simulink model "PV_wind_bat_DC_Microgrid"  (R2013a)
settings: Solver=ode23tb  StartTime=0  StopTime=3  RelTol=1e-3
undefined symbols (not defined in the file): c1, c2, c3, c4, c5, c6, DiscIntNeverNeededParam, fdesignblkfcn, gcbh, Hydride, Metal, Nickel
libraries: dspsigops x53, powerlib x33, powerlib_extras x6, electricdrivelib x1, dsparch4 x1, simulink x1
(part 1 of 2)
settings Model: Creator=cbhende  LastModifiedBy=user
settings SolverCC: ZeroCrossControl=DisableAll
settings DataIOCC: SaveFormat=StructureWithTime  SignalLoggingSaveFormat=ModelDataLogs  SaveOutput=off  SignalLogging=off  SaveTime=off
settings OptimizationCC: InlineParams=on  ExpressionDepthLimit=2147483647  InitFltsAndDblsToZero=on  EfficientFloat2IntCast=on
settings DebuggingCC: FcnCallInpInsideContextMsg=UseLocalSettings  StrictBusMsg=Warning
settings GRTTargetCC: CombineOutputUpdateFcns=off  GRTInterface=on

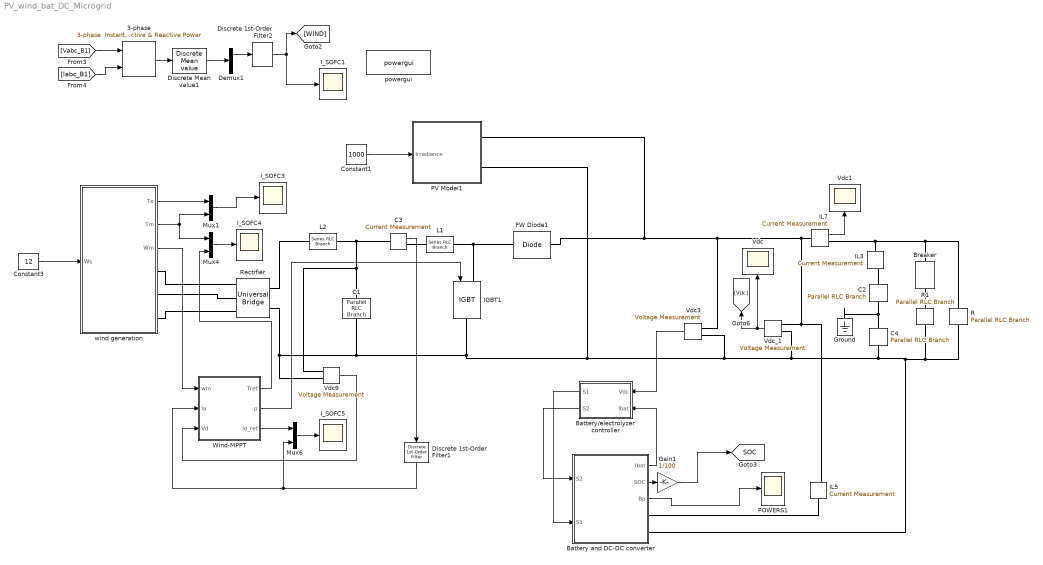
== system PV_wind_bat_DC_Microgrid ==
  "3-phase " : powerlib_extras/Measurements/3-phase  Instantaneous  Active & Reactive Power
  Battery and DC-DC converter : Subsystem
  Battery/electrolyzer controller : Subsystem
  Breaker : powerlib/Elements/Breaker  BreakerResistance=0.01  InitialState=0  SnubberResistance=1e6  SnubberCapacitance=inf  SwitchingTimes=[1 5]  External=off  Measurements=None  MoreParameters=off  NoBreakLoop=off
  C1 : powerlib/Elements/Parallel RLC Branch  LConnTagsString=a  RConnTagsString=__new0  BranchType=C  Resistance=1.0  Inductance=1.0  SetiL0=off  InitialCurrent=0  Capacitance=1000e-06  Setx0=off  InitialVoltage=0  Measurements=None
  C2 : powerlib/Elements/Parallel RLC Branch  LConnTagsString=a  RConnTagsString=__new0  BranchType=C  Resistance=1.0  Inductance=1.0  SetiL0=off  InitialCurrent=0  Capacitance=2200e-06*2  Setx0=off  InitialVoltage=0  Measurements=None
  C3 : powerlib/Measurements/Current Measurement  PhasorSimulation=off  OutputType=Complex  PSBequivalent=0
  C4 : powerlib/Elements/Parallel RLC Branch  LConnTagsString=a  RConnTagsString=__new0  BranchType=C  Resistance=1.0  Inductance=1.0  SetiL0=off  InitialCurrent=0  Capacitance=2200e-06*2  Setx0=off  InitialVoltage=0  Measurements=None
  Constant1 : Constant  Value=1000
  Constant3 : Constant  Value=12
  Demux1 : Demux  Outputs=2
  Discrete 1st-Order Filter1 : powerlib_extras/Discrete  Control Blocks/Discrete 1st-Order Filter  FilterType=Lowpass  Tc=100e-3  Ts=20e-6  Initialize=off  Vac_Init=[0.8 -25 60]  Vdc_Init=-0.4  PlotResponse=off  param1=[1 500 0.1]
  Discrete 1st-Order Filter2 : powerlib_extras/Discrete  Control Blocks/Discrete 1st-Order Filter  FilterType=Lowpass  Tc=100e-3  Ts=20e-6  Initialize=off  Vac_Init=[0.8 -25 60]  Vdc_Init=-0.4  PlotResponse=off  param1=[1 500 0.1]
  Discrete Mean value1 : powerlib_extras/Discrete Measurements/Discrete  Mean value  Freq=50  Vinit=0  Ts=20e-6
  FW Diode1 : powerlib/Power Electronics/Diode  Ron=0.01  Lon=0  Vf=0.8  IC=0  UseSnubber=off  Rs=100  Cs=0.1e-6  Measurements=off
  Gain1 : Gain  Gain=1/100
  Ground : powerlib/Elements/Ground  LConnTagsString=a
  IGBT1 : powerlib/Power Electronics/IGBT  Ron=0.001  Lon=0  Vf=1  Tf=1e-6  Tt=2e-6  IC=0  Rs=1e5  Cs=inf  Measurements=off
  IL3 : powerlib/Measurements/Current Measurement  PhasorSimulation=off  OutputType=Complex  PSBequivalent=0
  IL5 : powerlib/Measurements/Current Measurement  PhasorSimulation=off  OutputType=Complex  PSBequivalent=0
  IL7 : powerlib/Measurements/Current Measurement  PhasorSimulation=off  OutputType=Complex  PSBequivalent=0
  I_SOFC{1,3..5} (4 alike) : Scope
      I_SOFC1 settings: TimeRange=1.5  YMin=6213.5  YMax=6222  SaveName=w  SampleTime=100e-6
      I_SOFC3 settings: TimeRange=0.04  YMin=3400  YMax=3675  SaveName=Vdc  SampleInput=on  SampleTime=100e-6
      I_SOFC4 settings: TimeRange=0.04  YMin=3400  YMax=3675  SaveName=Vdc1  SampleInput=on  SampleTime=100e-6
      I_SOFC5 settings: TimeRange=0.04  YMin=3400  YMax=3675  SaveName=Vdc2  SampleInput=on  SampleTime=100e-6
  L1 : powerlib/Elements/Series RLC Branch  LConnTagsString=__new0  RConnTagsString=__new0  BranchType=L  Resistance=1.0  Inductance=2e-3  SetiL0=off  InitialCurrent=0  Capacitance=1.0  Setx0=off  InitialVoltage=0  Measurements=None
  L2 : powerlib/Elements/Series RLC Branch  LConnTagsString=__new0  RConnTagsString=__new0  BranchType=L  Resistance=1.0  Inductance=2e-3  SetiL0=off  InitialCurrent=0  Capacitance=1.0  Setx0=off  InitialVoltage=0  Measurements=None
  Mux1 : Mux  Inputs=2
  Mux4 : Mux  Inputs=2
  Mux6 : Mux  Inputs=2
  POWERS1 : Scope
      settings: TimeRange=1.5  YMin=-4410  YMax=-4260  SaveName=power1
  PV Model1 : Subsystem  mask{Isc=8.01, Voc=36.90, Im=7.10, Vm=30.3, ns=22}
      mask prompts: Isc "Short-Circuit Current"; Voc "Open-Circuit Voltage"; Im "Current at Pmax"; Vm "Voltage at Pmax"; ns "Number of Modules connected in series"
      mask init:
      | % calculation of PV module parameters
      | % limitation: constant temperature
      | Ns = round(Voc/0.61); % default number of cells in series
      | Vt = 26e-3; % thermal voltage
      | G = Isc/1000; % irradiation to short-circuit current gain
      | Vmpc = Vm/Ns; % cell voltage at rated Pmax
      | Vocc = Voc/Ns; % cell open-circuit voltage
      | Rmpp = Vmpc/Im; % cell load resistance at Pmax
      | %
      | Rp = 100*Vocc/Isc; % initial value for Rp
      | Vdm = Vocc; % initial value for Vdm
      | %
      | % iterative solution for model parameters: Io, Rs, Rp
      | for i=1:10
      | %
      |  Idm = Isc - Im - Vdm/Rp; % pn-junction (diode) current at MPP
      |  Io = (Isc-Vocc/Rp)/(exp(Vocc/Vt)-1); % pn-junction reverse saturation current
      |  Vdm = Vt*log(Idm/Io+1); % pn-junction (diode) voltage at MPP
      |  Rs = (Vdm-Vmpc)/Im; % cell series resistance
      |  Rd = (Rmpp - Rs)*Rp/(Rp-Rmpp+Rs); % diode incremental resistance at MPP
      |  Idm = Vt/Rd; % diode current at MPP based on incremental resistance
      |  Rp = Vdm/(Isc-Im-Idm); % cell parallel resistance
      | %
      | end
      | %
  R : powerlib/Elements/Parallel RLC Branch  LConnTagsString=a  RConnTagsString=__new0  BranchType=R  Resistance=400  Inductance=1.0  SetiL0=off  InitialCurrent=0  Capacitance=2200e-06*2  Setx0=off  InitialVoltage=0  Measurements=None
  R1 : powerlib/Elements/Parallel RLC Branch  LConnTagsString=a  RConnTagsString=__new0  BranchType=R  Resistance=200  Inductance=1.0  SetiL0=off  InitialCurrent=0  Capacitance=2200e-06*2  Setx0=off  InitialVoltage=0  Measurements=None
  Rectifier : powerlib/Power Electronics/Universal Bridge  Arms=3  SnubberResistance=100  SnubberCapacitance=0.1e-6  Device=Diodes  Ron=1e-3  Lon=0  ForwardVoltages="[  0.8  0.8  ]"  ForwardVoltage=.8  GTOparameters=[ 10e-6 , 20e-6 ]  IGBTparameters=[ 1e-6 , 2e-6 ]  Measurements=Device currents  Measurements_2=None  converterType=Rectifier
  Vdc : Scope
      settings: YMin=658  YMax=678  SaveName=V_dc  SampleInput=on  SampleTime=100e-6
  Vdc1 : Scope
      settings: YMin=658  YMax=677  SaveName=V_dc1  SampleInput=on  SampleTime=100e-6
  Vdc3 : powerlib/Measurements/Voltage Measurement  Tag=PoWeRsYsTeMmEaSuReMeNt  PhasorSimulation=off  OutputType=Magnitude  PSBequivalent=0
  Vdc9 : powerlib/Measurements/Voltage Measurement  Tag=PoWeRsYsTeMmEaSuReMeNt  PhasorSimulation=off  OutputType=Magnitude  PSBequivalent=0
  Vdc_1 : powerlib/Measurements/Voltage Measurement  Tag=PoWeRsYsTeMmEaSuReMeNt  PhasorSimulation=off  OutputType=Magnitude  PSBequivalent=0
  Wind-MPPT : Subsystem
  powergui : powerlib/powergui  SimulationMode=Discrete  SolverType=Tustin  SampleTime=20e-6  frequency=60  SPID=off  DisableSnubberDevices=off  DisableRonSwitches=off  DisableVfSwitches=off  SwTol=0  Interpol=off  DisplayEquations=off  frequencyindice=0  Pbase=100e6  ErrMax=1e-4  Iterations=50  UnitsV=kV  UnitsW=MW  FunctionMessages=off  echomessages=off  HookPort=off  EnableUseOfTLC=off  x0status=blocks  RestoreLinks=warning  ResistiveCurrentMeasurement=off  Frange=[0:2:500]  Ylog=off  Xlog=on  ShowGrid=off  save=off  variable=ZData  structure=psbbridges_str  ZoomFFT=on  StartTime=2.5  cycles=1  DisplayStyle=2  fundamental=50  FreqAxis=on  MaxFrequency=5000  frequencyindicesteady=1  RmsSteady=1  display=off  Ts=0  methode=off
  wind generation : Subsystem
  tag scope: SOC=global
  wires:
  Battery/electrolyzer controller/1(S1) -> Battery and DC-DC converter/2(S1)
  Battery/electrolyzer controller/2(S2) -> Battery and DC-DC converter/1(S2)
  Battery and DC-DC converter/1(Ibat) -> Battery/electrolyzer controller/2(Ibat)
  Battery and DC-DC converter/2(SOC) -> Gain1/1
  Vdc3/1 -> Battery/electrolyzer controller/1(Vdc)
  Vdc_1/1 -> Vdc/1, [Vdc]
  Battery and DC-DC converter/3(Bp) -> POWERS1/1
  Gain1/1 -> [SOC]
  Constant1/1 -> PV Model1/1(Irradiance)
  wind generation/2(Tm) -> Mux4/1, Mux1/2
  Wind-MPPT/1(Tref) -> Mux4/2
  wind generation/1(Te) -> Mux1/1
  wind generation/3(Wm) -> Wind-MPPT/1(wm)
  Constant3/1 -> wind generation/1(Ws)
  C3/1 -> Discrete 1st-Order Filter1/1
  Mux1/1 -> I_SOFC3/1
  Mux4/1 -> I_SOFC4/1
  Wind-MPPT/2(p) -> IGBT1/1
  Vdc9/1 -> Wind-MPPT/3(Vd)
  Discrete 1st-Order Filter1/1 -> Wind-MPPT/2(Ia), Mux6/2
  Mux6/1 -> I_SOFC5/1
  Wind-MPPT/3(Id_ref) -> Mux6/1
  [Vabc_B1] -> "3-phase "/1
  Discrete Mean value1/1 -> Demux1/1
  [Iabc_B1] -> "3-phase "/2
  "3-phase "/1 -> Discrete Mean value1/1
  Demux1/1 -> Discrete 1st-Order Filter2/1
  Discrete 1st-Order Filter2/1 -> [WIND], I_SOFC1/1
  IL7/1 -> Vdc1/1
  connections:
  IL3/RConn1 -- C2/LConn1
  IL5/RConn1 -- PV Model1/RConn1 -- FW Diode1/RConn1 -- Vdc3/LConn1 -- IL7/LConn1 -- Vdc_1/LConn1
  C1/RConn1 -- PV Model1/RConn2 -- R/RConn1 -- R1/RConn1 -- Battery and DC-DC converter/RConn2 -- C4/RConn1 -- Vdc_1/LConn2 -- Vdc3/LConn2 -- IGBT1/RConn1 -- Vdc9/LConn2 -- Rectifier/RConn2
  Battery and DC-DC converter/RConn1 -- IL5/LConn1
  IL7/RConn1 -- R/LConn1 -- Breaker/LConn1 -- IL3/LConn1
  C4/LConn1 -- Ground/LConn1 -- C2/RConn1
  C3/LConn1 -- L2/RConn1 -- Vdc9/LConn1 -- C1/LConn1
  L1/RConn1 -- FW Diode1/LConn1 -- IGBT1/LConn1
  wind generation/RConn2 -- Rectifier/LConn2
  wind generation/RConn1 -- Rectifier/LConn1
  wind generation/RConn3 -- Rectifier/LConn3
  Rectifier/RConn1 -- L2/LConn1
  C3/RConn1 -- L1/LConn1
  R1/LConn1 -- Breaker/RConn1

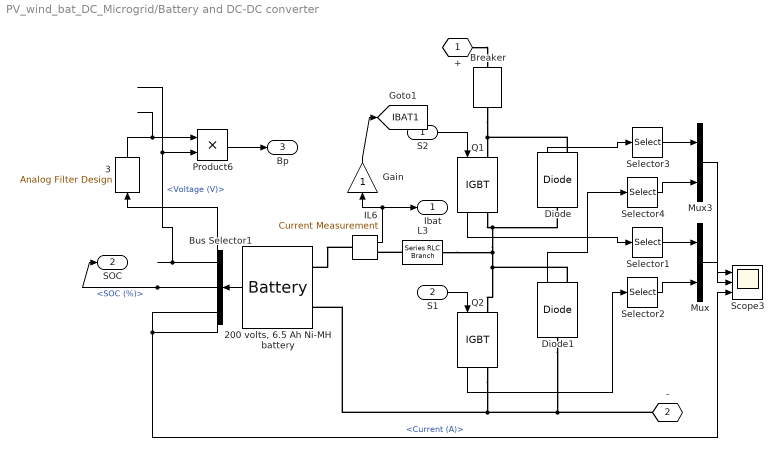
== system PV_wind_bat_DC_Microgrid/Battery and DC-DC converter ==
  S2 : Inport
  S1 : Inport  Port=2
  "200 volts, 6.5 Ah Ni-MH battery " : electricdrivelib/Extra Sources/Battery  BatType=Nickel-Metal-Hydride  ShowDetailedParameters=off  NomV=300  NomQ=50  SOC=60  PresetModel=on  MaxQ=53.8462  FullV=353.3898  Dis_rate=10  R=0.06  Normal_OP=48.0769  expZone="[325.4237            10]"  Dis_Char=off  current=[6.5 13 32.5]  Units=Time  Batt_Tr=30
  3 : dsparch4/Analog Filter Design  method=Butterworth  filttype=Lowpass  N=8  Wlo=pi*50  Whi=80  Rp=2  Rs=40
  Breaker : powerlib/Elements/Breaker  BreakerResistance=0.01  InitialState=1  SnubberResistance=1e6  SnubberCapacitance=inf  SwitchingTimes=[15 ]  External=off  Measurements=None  MoreParameters=off  NoBreakLoop=off
  Bus Selector1 : BusSelector  OutputSignals=Voltage (V),SOC (%),Current (A)
  Diode : powerlib/Power Electronics/Diode  Ron=0.001  Lon=0  Vf=0.8  IC=0  UseSnubber=off  Rs=500  Cs=250e-9  Measurements=on
  Diode1 : powerlib/Power Electronics/Diode  Ron=0.001  Lon=0  Vf=0.8  IC=0  UseSnubber=off  Rs=500  Cs=250e-9  Measurements=on
  Gain : Gain
  IL6 : powerlib/Measurements/Current Measurement  PhasorSimulation=off  OutputType=Complex  PSBequivalent=0
  L3 : powerlib/Elements/Series RLC Branch  LConnTagsString=__new0  RConnTagsString=__new0  BranchType=L  Resistance=1.0  Inductance=5e-3  SetiL0=off  InitialCurrent=0  Capacitance=1.0  Setx0=off  InitialVoltage=0  Measurements=None
  Mux : Mux  Inputs=2
  Mux3 : Mux  Inputs=2
  Product6 : Product  RndMeth=Zero
  Q1 : powerlib/Power Electronics/IGBT  Ron=0.001  Lon=0  Vf=1  Tf=1e-6  Tt=2e-6  IC=0  Rs=1e5  Cs=inf  Measurements=on
  Q2 : powerlib/Power Electronics/IGBT  Ron=0.001  Lon=0  Vf=1  Tf=1e-6  Tt=2e-6  IC=0  Rs=1e5  Cs=inf  Measurements=on
  Scope3 : Scope  NumInputPorts=3
      settings: TimeRange=0.1  YMin=0~0~-36  YMax=37.5~35~-23  SaveName=V2X  SampleInput=on  SampleTime=10e-6
  Selector{1..4} (4 alike) : Selector  InputPortWidth=2  IndexOptions=Index vector (dialog)  Indices=1  OutputSizes=1
  + : PMIOPort  Tag=PMCPort  Port=1  Side=Right
  - : PMIOPort  Tag=PMCPort  Port=2  Side=Right
  Ibat : Outport
  SOC : Outport  Port=2
  Bp : Outport  Port=3
  tag scope: IBAT1=global
  wires:
  "200 volts, 6.5 Ah Ni-MH battery "/1 -> Bus Selector1/1
  Bus Selector1/1 -> Product6/2  "<Voltage (V)>"
  Bus Selector1/2 -> SOC/1  "<SOC (%)>"
  Bus Selector1/3 -> Scope3/3, 3/1  "<Current (A)>"
  Product6/1 -> Bp/1
  Q1/1 -> Selector1/1
  Q2/1 -> Selector2/1
  Selector1/1 -> Mux/1
  Selector2/1 -> Mux/2
  Selector3/1 -> Mux3/1
  Selector4/1 -> Mux3/2
  Diode/1 -> Selector3/1
  Diode1/1 -> Selector4/1
  Mux/1 -> Scope3/1
  Mux3/1 -> Scope3/2
  S2/1 -> Q1/1
  S1/1 -> Q2/1
  IL6/1 -> Ibat/1, Gain/1
  3/1 -> Product6/1
  Gain/1 -> [IBAT1]
  connections:
  IL6/LConn1 -- "200 volts, 6.5 Ah Ni-MH battery "/LConn1
  "200 volts, 6.5 Ah Ni-MH battery "/LConn2 -- Q2/RConn1 -- -/RConn1 -- Diode1/LConn1
  +/RConn1 -- Breaker/LConn1
  Breaker/RConn1 -- Diode/RConn1 -- Q1/LConn1
  Q2/LConn1 -- Diode1/RConn1 -- L3/RConn1 -- Diode/LConn1 -- Q1/RConn1
  L3/LConn1 -- IL6/RConn1

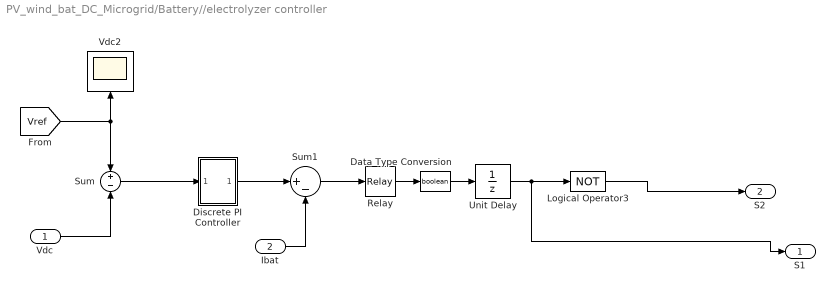
== system PV_wind_bat_DC_Microgrid/Battery//electrolyzer controller ==
  Vdc : Inport
  Ibat : Inport  Port=2
  Data Type Conversion : DataTypeConversion  OutDataTypeStr=boolean  RndMeth=Simplest  SaturateOnIntegerOverflow=on
  Discrete PI Controller : Subsystem  AncestorBlock=|  DialogController=POWERSYS.PowerSysDialog  mask(Discrete PI Controller){Kp=3, Ki=180, Par_Limits=[100  -100], Init=0, Ts=20e-6}
      | powerlib_extras/Discrete 
      | Control Blocks/Discrete
      | PI Controller
      mask prompts: Kp "Proportional gain (Kp):"; Ki "Integral gain (Ki):"; Par_Limits "Output limits: [ Upper   Lower ]"; Init "Output initial value:"; Ts "Sample time:"
      mask help: This block implements a discrete PI controller.
      mask init:
      | UpperLimit=Par_Limits(1);
      | LowerLimit=Par_Limits(2);
      | power_initmask();
      mask Help: This block is part of a subset of blocks in the Extras library that does not have documentation associated with it, other than the block mask description.
      mask Display: disp('PI');
  Logical Operator3 : Logic  Operator=NOT
  Relay : Relay  OnSwitchValue=1  OffSwitchValue=-1  OutDataTypeStr=Inherit: Inherit via back propagation
  Sum : Sum  Inputs=+-  SaturateOnIntegerOverflow=on  InputSameDT=on  OutDataTypeStr=Inherit: Same as first input
  Sum1 : Sum  Inputs=|+-  InputSameDT=on
  Unit Delay : UnitDelay  SampleTime=-1
  Vdc2 : Scope
      settings: YMin=654.997  YMax=655  SaveName=V_dc3  SampleInput=on  SampleTime=100e-6
  S1 : Outport
  S2 : Outport  Port=2
  wires:
  Vdc/1 -> Sum/2
  Logical Operator3/1 -> S2/1
  Discrete PI Controller/1(Out) -> Sum1/1
  Sum/1 -> Discrete PI Controller/1(Error)
  Relay/1 -> Data Type Conversion/1
  Ibat/1 -> Sum1/2
  Sum1/1 -> Relay/1
  Data Type Conversion/1 -> Unit Delay/1
  [Vref] -> Sum/1, Vdc2/1
  Unit Delay/1 -> S1/1, Logical Operator3/1

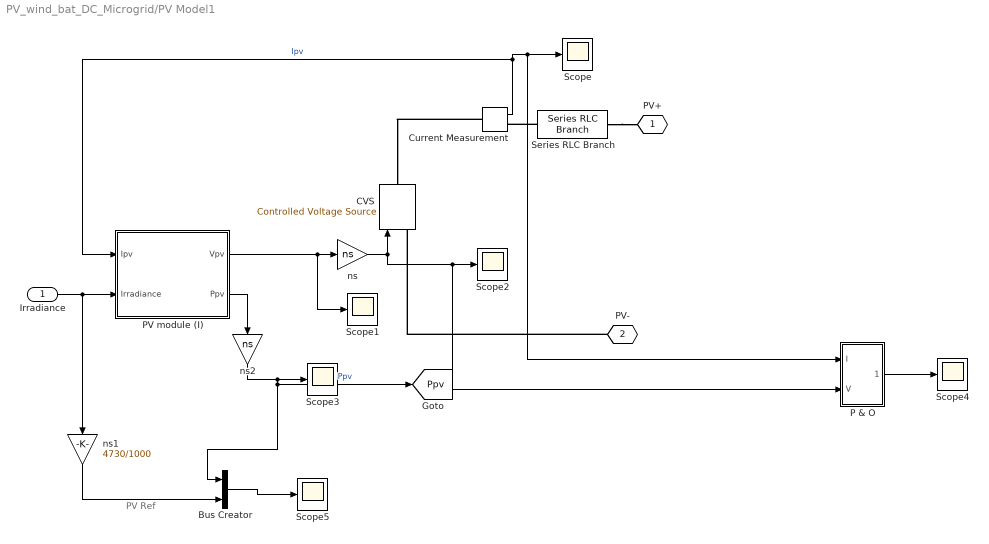
== system PV_wind_bat_DC_Microgrid/PV Model1 ==
  note: PV Ref
  Irradiance : Inport
  Bus Creator : BusCreator  Inputs=2
  CVS : powerlib/Electrical Sources/Controlled Voltage Source  Initialize=on  Source_Type=DC  Amplitude=0  Phase=0  Frequency=0  Measurements=None
  Current Measurement : powerlib/Measurements/Current Measurement  PhasorSimulation=off  OutputType=Complex  PSBequivalent=0
  P & O : Subsystem
  PV module (I) : Subsystem
  Scope{,1..5} (6 alike) : Scope
      Scope settings: YMin=3.3  YMax=3.355
      Scope1 settings: SaveName=ScopeData2
      Scope2 settings: YMin=653  YMax=668  SaveName=ScopeData3
      Scope3 settings: YMin=4645  YMax=4695  SaveName=ScopeData4
      Scope4 settings: YMin=609.9  YMax=674.1  SaveName=ScopeData28
      Scope5 settings: YMin=4710  YMax=4733  SaveName=ScopeData42
  Series RLC Branch : powerlib/Elements/Series RLC Branch  LConnTagsString=__new0  RConnTagsString=__new0  BranchType=R  Resistance=0.00001  Inductance=1e-3  SetiL0=off  InitialCurrent=0  Capacitance=1e-6  Setx0=off  InitialVoltage=0  Measurements=None
  ns : Gain  Gain=ns
  ns1 : Gain  Gain=4730/1000
  ns2 : Gain  Gain=ns
  PV+ : PMIOPort  Tag=PMCPort  Port=1  Side=Right
  PV- : PMIOPort  Tag=PMCPort  Port=2  Side=Right
  tag scope: Ppv=global
  wires:
  ns2/1 -> [Ppv], Bus Creator/1, Scope3/1  "Ppv"
  ns/1 -> CVS/1, Scope2/1, P & O/2(V)
  PV module (I)/2(Ppv) -> ns2/1
  Irradiance/1 -> PV module (I)/2(Irradiance), ns1/1
  Current Measurement/1 -> PV module (I)/1(Ipv), Scope/1, P & O/1(I)  "Ipv"
  PV module (I)/1(Vpv) -> Scope1/1, ns/1
  P & O/1(Vref) -> Scope4/1
  ns1/1 -> Bus Creator/2
  Bus Creator/1 -> Scope5/1
  connections:
  Series RLC Branch/LConn1 -- Current Measurement/RConn1
  Current Measurement/LConn1 -- CVS/RConn1
  PV-/RConn1 -- CVS/LConn1
  Series RLC Branch/RConn1 -- PV+/RConn1

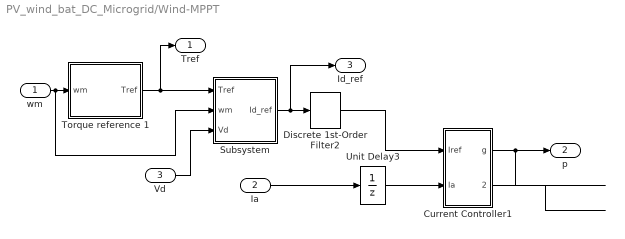
== system PV_wind_bat_DC_Microgrid/Wind-MPPT ==
  wm : Inport
  Ia : Inport  Port=2
  Vd : Inport  Port=3
  Current Controller1 : Subsystem  mask{h=0.1}
      mask prompts: h "Hysteresis band (A)"
      mask help: Hysteresis Current Controller
      mask Display: plot(0,0,100,100,[45,45],[35,65],[55,55],[35,65],[45,65],[65,65],[35,55],[35,35])
  Discrete 1st-Order Filter2 : powerlib_extras/Discrete  Control Blocks/Discrete 1st-Order Filter  FilterType=Lowpass  Tc=100e-3  Ts=20e-6  Initialize=off  Vac_Init=[0.8 -25 60]  Vdc_Init=-0.4  PlotResponse=off  param1=[1 500 0.1]
  Subsystem : Subsystem
  Torque reference 1 : Subsystem
  Unit Delay3 : UnitDelay  SampleTime=-1
  Tref : Outport
  p : Outport  Port=2
  Id_ref : Outport  Port=3
  wires:
  Unit Delay3/1 -> Current Controller1/2(Ia)
  Torque reference 1/1(Tref) -> Tref/1, Subsystem/1(Tref)
  Subsystem/1(Id_ref) -> Discrete 1st-Order Filter2/1, Id_ref/1
  Discrete 1st-Order Filter2/1 -> Current Controller1/1(Iref)
  Current Controller1/1(g) -> p/1
  wm/1 -> Torque reference 1/1(wm), Subsystem/2(wm)
  Vd/1 -> Subsystem/3(Vd)
  Ia/1 -> Unit Delay3/1
  Current Controller1/2(error1) -> ?

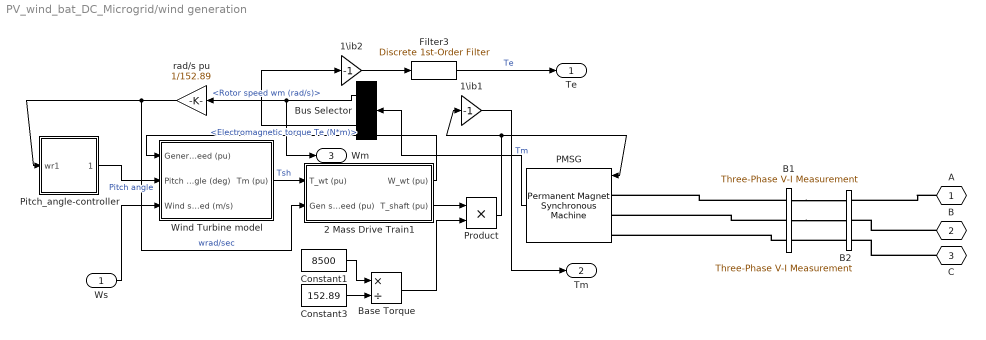
== system PV_wind_bat_DC_Microgrid/wind generation ==
  Ws : Inport
  1\ib1 : Gain  Gain=-1  SaturateOnIntegerOverflow=on  OutDataTypeStr=Inherit: Same as input  ParamDataTypeStr=Inherit: Same as input
  1\ib2 : Gain  Gain=-1  SaturateOnIntegerOverflow=on  OutDataTypeStr=Inherit: Same as input  ParamDataTypeStr=Inherit: Same as input
  2 Mass Drive Train1 : Subsystem
  B1 : powerlib/Measurements/Three-Phase V-I Measurement  VoltageMeasurement=phase-to-ground  SetLabelV=on  LabelV=Vabc_B1  Vpu=off  VpuLL=off  CurrentMeasurement=yes  SetLabelI=on  LabelI=Iabc_B1  Ipu=off  Pbase=100e6  Vbase=500e3  OutputType=Magnitude  PhasorSimulation=off  PSBequivalent=0
  "B2 " : powerlib/Measurements/Three-Phase V-I Measurement  VoltageMeasurement=no  SetLabelV=on  LabelV=Vabc_B2  Vpu=off  VpuLL=off  CurrentMeasurement=no  SetLabelI=on  LabelI=Iabc_B2  Ipu=off  Pbase=100e6  Vbase=500e3  OutputType=Magnitude  PhasorSimulation=off  PSBequivalent=0
  Base Torque : Product  Inputs=*/  RndMeth=Zero
  Bus Selector : BusSelector  OutputSignals=Rotor speed wm (rad/s),Electromagnetic torque Te (N*m)
  Constant1 : Constant  Value=8500
  Constant3 : Constant  Value=152.89
  Filter3 : powerlib_extras/Discrete  Control Blocks/Discrete 1st-Order Filter  FilterType=Lowpass  Tc=1e-3  Ts=20e-6  Initialize=off  Vac_Init=[0.8 -25 60]  Vdc_Init=-0.4  PlotResponse=off  param1=[1 500 0.1]
  PMSG : powerlib/Machines/Permanent Magnet Synchronous Machine  NbPhases=3  FluxDistribution=Sinusoidal  RotorType=Round  MechanicalLoad=Torque Tm  PresetModel=No  ShowDetailedParameters=on  Resistance=0.425  Inductance=8.5e-3  dqInductances=[0.0082 0.0082]  La=0.000835  MachineConstant=Flux linkage established by magnets (V.s)  Flux=0.433  VoltageCst=392.6876  TorqueCst=3.2475  Flat=120  Mechanical=[0.01197 0.001189 5]  PolePairs=5  InitialConditions=[0,0, 0,0]  InitialConditions5ph=[0 0 0 0 0 0]  TsPowergui=0  TsBlock=-1  RefAngle=90 degrees behind phase A axis (modified Park)
  Pitch_angle-controller : Subsystem
  Product : Product  RndMeth=Zero
  Wind Turbine model : Subsystem  AncestorBlock=DRlib/Wind Generation/Wind Turbine  DialogController=POWERSYS.PowerSysDialog  mask(Wind Turbine){Pnom=8.5e3, Pelec_base=8.5e3/0.9, wind_base=12, P_wind_base=0.8, speed_nom=1, pitch_angle=0, DisplayTurbChar=off, c1_c6=[0.51763          116          0.4            5           21     0.006795], cp_nom=0.48, lambda_nom=8.1}
      mask prompts: Pnom "Nominal mechanical output power (W):"; Pelec_base "Base power of the electrical generator (VA):"; wind_base "Base wind speed (m/s):"; P_wind_base "Maximum power at base wind speed (pu of nominal mechanical power):"; speed_nom "Base rotational speed (p.u. of base generator speed):"; pitch_angle "Pitch angle beta to display wind-turbine power characteristics (beta >=0)  (deg):"; DisplayTurbChar "Display wind turbine power characteristics"
      mask help:
      | This block implements a variable pitch wind turbine model. The performance coefficient Cp of the turbine is the mechanical output power of the turbine divided by wind power and a function of wind speed, rotational speed, and pitch angle (beta). Cp reaches its maximum value at zero beta. Select the wind-turbine power characteristics display to plot the turbine characteristics at the specified pitch angle.
      |
      | The first input is the generator speed in per unit of the generator base speed. For a synchronous or asynchronous generator, the base speed is the synchronous speed. For a permanent-magnet generator, the base speed is defined as the speed producing nominal voltage at  no load. The second input is the blade pitch angle (beta) in degrees. The third input is the wind speed in m/s.
      |
      | The output is the torque applied to the generator shaft in per unit of the generator ratings.
      |
      | The turbine inertia must be added to the generator inertia.
      mask init:
      | %Wind turbine typical characteristic data
      | %c2=116;c3=0.4;c4=5;c5=21;
      | %Computation of c1 and c6 for lambda_nom et cpmax
      | %lambda_nom=8.1;
      | %cp_max=0.48;
      | %cp_nom=cp_max;
      | 
      | %lambda_i_nom=1/(1/lambda_nom-0.035);
      | %k_nom=-(c2*c5/lambda_i_nom-c4*c5-c2)*exp(-c5/lambda_i_nom)/lambda_nom^2;
      | %c1=cp_max/((c2/lambda_i_nom-c4)*exp(-c5/lambda_i_nom)+k_nom*lambda_nom);
      | %c6=k_nom*c1;
      | power_initmask();
      mask Help: web(psbhelp);
      mask Callback Pnom:
      | ParVisible={'on','on','on','on','on','on','on','off','off','off',};
      | set_param(gcb,'MaskVisibilities',ParVisible);
      | c1_c6=str2num(get_param(gcb,'c1_c6'));
      | c1=c1_c6(1);c2=c1_c6(2);c3=c1_c6(3);c4=c1_c6(4);c5=c1_c6(5);c6=c1_c6(6);
      mask Callback DisplayTurbChar:
      | DisplayTurbChar=get_param(gcb,'DisplayTurbChar');
      | 
      | if strcmp(DisplayTurbChar,'on')
      |     fig_num=figure;
      | 	clf(fig_num);
      | 	[speed_nom,wind_base,P_wind_base,pitch_angle]=getSPSmaskvalues(gcb,{'speed_nom','wind_base','P_wind_base','pitch_angle'});
      | 	[c1_c6,lambda_nom,cp_nom]=getSPSmaskvalues(gcb,{'c1_c6','lambda_nom','cp_nom'});
      | 	c1=c1_c6(1);c2=c1_c6(2);c3=c1_c6(3);c4=c1_c6(4);c5=c1_c6(5);c6=c1_c6(6);
      | 
      | 	%Wind turbine typical characteristic data
      |     %c2=116;c3=0.4;c4=5;c5=21;
      |     %Computation of c1 and c6 for lambda_nom et cpmax
      |     %lambda_nom=8.1;
      |     %cp_max=0.48;
      |     %cp_nom=cp_max;
      | 
      |     %lambda_i_nom=1/(1/lambda_nom-0.035);
      |     %k_nom=-(c2*c5/lambda_i_nom-c4*c5-c2)*exp(-c5/lambda_i_nom)/lambda_nom^2;
      |     %c1=cp_max/((c2/lambda_i_nom-c4)*exp(-c5/lambda_i_nom)+k_nom*lambda_nom);
      |     %c6=k_nom*c1;
      | 
      | 	wr_elec_pu=1e-3:0.01:1.5;;
      |     wr_mec_pu=wr_elec_pu/speed_nom;
      |     wind_max=ceil((1.2/P_wind_base)^(1/3)*wind_base);
      |     wind_min=round(((0.1)/P_wind_base)^(1/3)*wind_base);
      |     wind1=wind_min:(wind_base-wind_min)/5:wind_base;
      |     wind2=wind_base+(wind_base-wind_min)/5:(wind_base-wind_min)/5:wind_max;
      |     wind_pu=[wind1 wind2]/wind_base;
      | 
      |     for k=1:length(wind_pu)
      |         for i=1:length(wr_mec_pu);
      |             lambda_pu=wr_mec_pu(i)/wind_pu(k);
      |             lambda=lambda_pu*lambda_nom;
      |             lambda_i=1/(1/(lambda+0.08*pitch_angle)-0.035/(pitch_angle^3+1));
      |             cp=c1*(c2/lambda_i-c3*pitch_angle-c4)*exp(-c5/lambda_i)+c6*lambda;
      |             cp_pu=cp/cp_nom;
      |             Pwind_pu(k,i)=wind_pu(k)^3*cp_pu*P_wind_base;
      |         end
      |     end
      |     for k=1:length(wind_pu)
      |         plot(wr_elec_pu,Pwind_pu(k,:))
      |         hold on
      |     end
      | 
      |     plot([speed_nom,speed_nom,0],[0,P_wind_base,P_wind_base],'r--')
      |     text(speed_nom+0.01,0+0.05,sprintf('%0.4g pu',speed_nom))
      |     text(0.01,P_wind_base+0.05,sprintf('Max. power at base wind speed (%0.4g m/s) and beta = 0 deg',wind_base))
      |     for i=1:length(wind_pu),
      |         p_max(i)=max(Pwind_pu(i,:));
      |         speed(i)=wr_elec_pu(find(Pwind_pu(i,:)==p_max(i)));
      |         text(speed(i),p_max(i),sprintf('%0.4g m/s',wind_pu(i)*wind_base))
      |     end
      |     plot([0 max(wr_elec_pu)],[0 0],'--')
      | 
      |     xlabel('Turbine speed (pu of nominal generator speed)')
      |     ylabel('Turbine output power (pu of nominal mechanical power)')
      |     title(sprintf('Turbine Power Characteristics (Pitch angle beta = %0.4g deg)',pitch_angle))
      |     axis([0 max(wr_elec_pu) min(Pwind_pu(1,:)) max(P_wind_base+0.1,max(wind_pu)^3*P_wind_base+0.1)])
      |     set_param(gcb,'DisplayTurbChar','off')
      | end
      mask Display: disp('');
  rad/s pu : Gain  Gain=1/152.89  SaturateOnIntegerOverflow=on  OutDataTypeStr=Inherit: Same as input  ParamDataTypeStr=Inherit: Same as input
  A : PMIOPort  Tag=PMCPort  Port=1  Side=Right
  B : PMIOPort  Tag=PMCPort  Port=2  Side=Right
  C : PMIOPort  Tag=PMCPort  Port=3  Side=Right
  Te : Outport
  Tm : Outport  Port=2
  Wm : Outport  Port=3
  wires:
  Bus Selector/1 -> rad/s pu/1, Wm/1  "<Rotor speed wm (rad/s)>"
  rad/s pu/1 -> Pitch_angle-controller/1(wr1), 2 Mass Drive Train1/2(Gen speed (pu))  "wrad/sec"
  1\ib2/1 -> Filter3/1
  Filter3/1 -> Te/1  "Te"
  Product/1 -> PMSG/1, 1\ib1/1
  Pitch_angle-controller/1(Pitch_angle1) -> Wind Turbine model/2(Pitch angle (deg))  "Pitch angle"
  Constant1/1 -> Base Torque/1
  Constant3/1 -> Base Torque/2
  PMSG/1 -> Bus Selector/1
  Bus Selector/2 -> 1\ib2/1  "<Electromagnetic torque Te (N*m)>"
  Ws/1 -> Wind Turbine model/3(Wind speed (m/s))
  Wind Turbine model/1(Tm (pu)) -> 2 Mass Drive Train1/1(T_wt (pu))  "Tsh"
  Base Torque/1 -> Product/2
  2 Mass Drive Train1/1(W_wt (pu)) -> Wind Turbine model/1(Generator speed (pu))
  2 Mass Drive Train1/2(T_shaft (pu)) -> Product/1
  1\ib1/1 -> Tm/1  "Tm"
  connections:
  B1/LConn2 -- PMSG/LConn2
  B1/LConn3 -- PMSG/LConn3
  B1/RConn1 -- "B2 "/LConn1
  B1/RConn2 -- "B2 "/LConn2
  "B2 "/LConn3 -- B1/RConn3
  A/RConn1 -- "B2 "/RConn1
  B/RConn1 -- "B2 "/RConn2
  C/RConn1 -- "B2 "/RConn3
  B1/LConn1 -- PMSG/LConn1

== system PV_wind_bat_DC_Microgrid/Battery//electrolyzer controller/Discrete PI Controller ==
  Error : Inport
  Discrete-Time Integrator : DiscreteIntegrator  InitialCondition=Init  SampleTime=Ts  LimitOutput=on  UpperSaturationLimit=UpperLimit  LowerSaturationLimit=LowerLimit  ICPrevOutput=DiscIntNeverNeededParam  ICPrevScaledInput=DiscIntNeverNeededParam
  Kp4 : Gain  Gain=Kp  SaturateOnIntegerOverflow=on  OutDataTypeStr=Inherit: Same as input  ParamDataTypeStr=Inherit: Same as input
  Kp5 : Gain  Gain=Ki  SaturateOnIntegerOverflow=on  OutDataTypeStr=Inherit: Same as input  ParamDataTypeStr=Inherit: Same as input
  Saturation2 : Saturate  UpperLimit=UpperLimit  LowerLimit=LowerLimit
  Sum6 : Sum  SaturateOnIntegerOverflow=on  InputSameDT=on  OutDataTypeStr=Inherit: Same as first input
  Out : Outport  InitialOutput=0
  wires:
  Saturation2/1 -> Out/1
  Discrete-Time Integrator/1 -> Sum6/2
  Kp4/1 -> Sum6/1
  Kp5/1 -> Discrete-Time Integrator/1
  Sum6/1 -> Saturation2/1
  Error/1 -> Kp5/1, Kp4/1

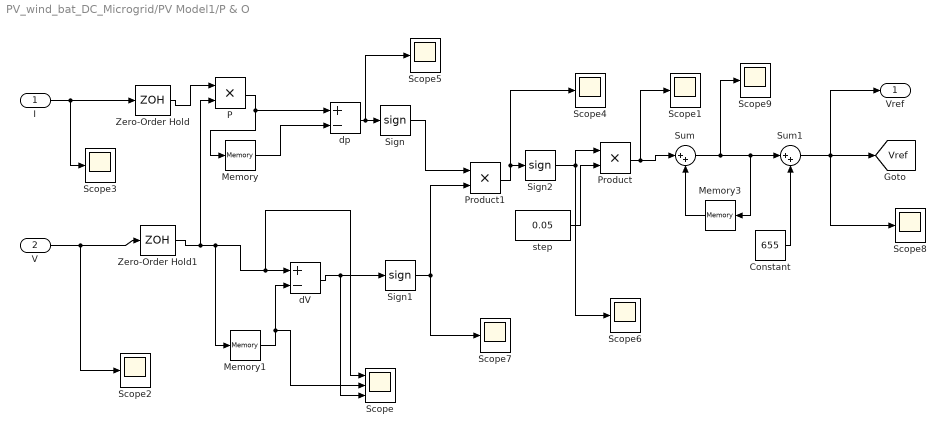
== system PV_wind_bat_DC_Microgrid/PV Model1/P & O ==
  I : Inport
  V : Inport  Port=2
  Constant : Constant  Value=655
  Memory : Memory  InheritSampleTime=on
  Memory1 : Memory  InheritSampleTime=on
  Memory3 : Memory  InheritSampleTime=on
  P : Product  RndMeth=Zero
  Product : Product  RndMeth=Zero
  Product1 : Product  RndMeth=Zero
  Scope : Scope  NumInputPorts=3
      settings: YMin=29.1717~29.1717~1e-006  YMax=32.2424~32.2424~1.7e-005
  Scope{1..9} (9 alike) : Scope
      Scope1 settings: YMin=-0.0005  YMax=0.0005  SaveName=ScopeData34
      Scope2 settings: YMin=-11  YMax=10  SaveName=ScopeData35
      Scope3 settings: YMin=-11  YMax=10  SaveName=ScopeData36
      Scope4 settings: YMin=-11  YMax=10  SaveName=ScopeData37
      Scope5 settings: YMin=-11  YMax=10
      Scope6 settings: YMin=-11  YMax=10  SaveName=ScopeData38
      Scope7 settings: YMin=-11  YMax=10  SaveName=ScopeData39
      Scope8 settings: YMin=655  YMax=668  SaveName=ScopeData40
      Scope9 settings: YMin=-7.5  YMax=2.5  SaveName=ScopeData41
  Sign : Signum
  Sign1 : Signum
  Sign2 : Signum
  Sum : Sum  Inputs=|++
  Sum1 : Sum  Inputs=|++
  Zero-Order Hold : ZeroOrderHold  SampleTime=0.002
  Zero-Order Hold1 : ZeroOrderHold  SampleTime=0.002
  dV : Sum  Inputs=+-
  dp : Sum  Inputs=+-
  step : Constant  Value=0.05
  Vref : Outport
  tag scope: Vref=global
  wires:
  Memory1/1 -> dV/2, Scope/2
  Memory/1 -> dp/2
  V/1 -> Zero-Order Hold1/1, Scope2/1
  dV/1 -> Sign1/1, Scope/3
  step/1 -> Product/2
  Product/1 -> Sum/1, Scope1/1
  Sign/1 -> Product1/1
  Sign1/1 -> Product1/2, Scope7/1
  Product1/1 -> Sign2/1, Scope4/1
  I/1 -> Zero-Order Hold/1, Scope3/1
  Zero-Order Hold1/1 -> P/2, dV/1, Scope/1, Memory1/1
  Zero-Order Hold/1 -> P/1
  P/1 -> Memory/1, dp/1
  dp/1 -> Sign/1, Scope5/1
  Sign2/1 -> Product/1, Scope6/1
  Sum/1 -> Memory3/1, Sum1/1, Scope9/1
  Memory3/1 -> Sum/2
  Sum1/1 -> [Vref], Vref/1, Scope8/1
  Constant/1 -> Sum1/2

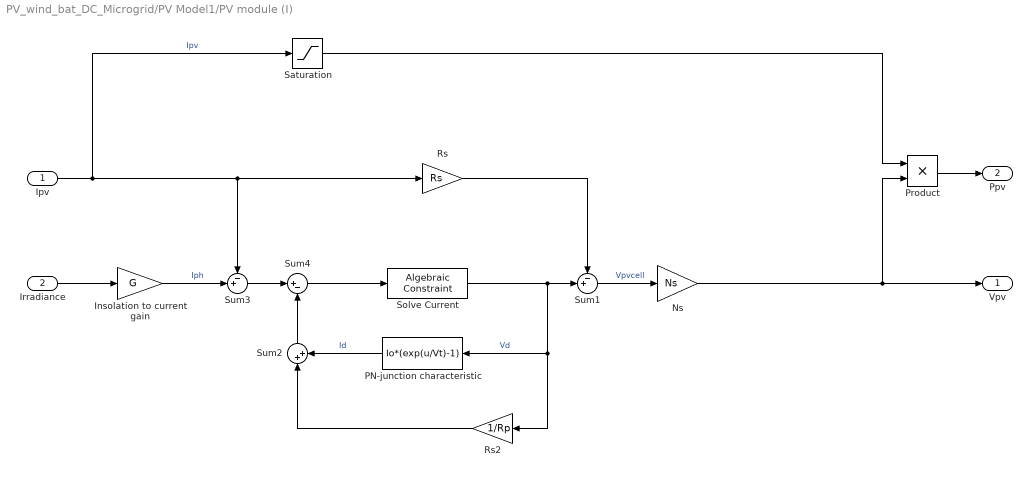
== system PV_wind_bat_DC_Microgrid/PV Model1/PV module (I) ==
  Ipv : Inport
  Irradiance : Inport  Port=2
  Insolation to current gain : Gain  Gain=G
  Ns : Gain  Gain=Ns
  PN-junction characteristic : Fcn  Expr=Io*(exp(u/Vt)-1)
  Product : Product  RndMeth=Zero
  Rs : Gain  Gain=Rs
  Rs2 : Gain  Gain=1/Rp
  Saturation : Saturate  UpperLimit=inf  LowerLimit=0
  Solve Current : simulink/Math Operations/Algebraic Constraint  z0=1.99
  Sum1 : Sum  Inputs=-+|
  Sum2 : Sum  Inputs=|++
  Sum3 : Sum  Inputs=-+|
  Sum4 : Sum  Inputs=|+-
  Vpv : Outport
  Ppv : Outport  Port=2
  wires:
  PN-junction characteristic/1 -> Sum2/2  "Id"
  Sum3/1 -> Sum4/1
  Saturation/1 -> Product/1
  Ns/1 -> Product/2, Vpv/1
  Rs/1 -> Sum1/1
  Sum1/1 -> Ns/1  "Vpvcell"
  Solve Current/1 -> Sum1/2, PN-junction characteristic/1, Rs2/1  "Vd"
  Sum4/1 -> Solve Current/1
  Product/1 -> Ppv/1
  Ipv/1 -> Rs/1, Sum3/1, Saturation/1  "Ipv"
  Insolation to current gain/1 -> Sum3/2  "Iph"
  Irradiance/1 -> Insolation to current gain/1
  Rs2/1 -> Sum2/1
  Sum2/1 -> Sum4/2

== system PV_wind_bat_DC_Microgrid/Wind-MPPT/Current Controller1 ==
  Iref : Inport
  Ia : Inport  Port=2
  Relay : Relay  OnSwitchValue=h/2  OffSwitchValue=-h/2
  Sum1 : Sum  Inputs=-+  SaturateOnIntegerOverflow=on  InputSameDT=on  OutDataTypeStr=Inherit: Same as first input
  g : Outport  InitialOutput=0
  error1 : Outport  Port=2  InitialOutput=0
  wires:
  Relay/1 -> g/1
  Ia/1 -> Sum1/1
  Iref/1 -> Sum1/2
  Sum1/1 -> Relay/1, error1/1

== system PV_wind_bat_DC_Microgrid/Wind-MPPT/Subsystem ==
  Tref : Inport
  wm : Inport  Port=2
  Vd : Inport  Port=3
  Avoid division by zero : Saturate  UpperLimit=1e6  LowerLimit=1e-6
  Base Torque1 : Product  Inputs=*/  RndMeth=Zero
  Product1 : Product  RndMeth=Zero
  Id_ref : Outport
  wires:
  Product1/1 -> Base Torque1/1
  Avoid division by zero/1 -> Base Torque1/2
  Tref/1 -> Product1/1
  wm/1 -> Product1/2
  Base Torque1/1 -> Id_ref/1
  Vd/1 -> Avoid division by zero/1

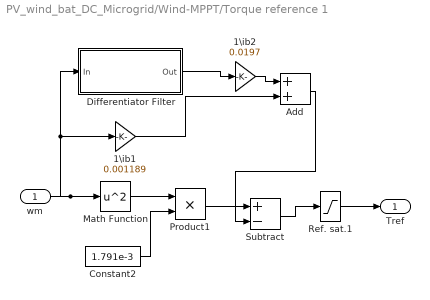
== system PV_wind_bat_DC_Microgrid/Wind-MPPT/Torque reference 1 ==
  wm : Inport
  1\ib1 : Gain  Gain=0.001189  SaturateOnIntegerOverflow=on  OutDataTypeStr=Inherit: Same as input  ParamDataTypeStr=Inherit: Same as input
  1\ib2 : Gain  Gain=0.0197  SaturateOnIntegerOverflow=on  OutDataTypeStr=Inherit: Same as input  ParamDataTypeStr=Inherit: Same as input
  Add : Sum
  Constant2 : Constant  Value=1.791e-3
  Differentiator Filter : Subsystem  DialogController=fdesignblkfcn  InitFcn=fdesignblkfcn(gcbh, {'InitFcn'});  mask(Differentiator Filter){}
      mask help: Design a differentiator filter
      settings: CopyFcn=fdesignblkfcn(gcbh, {'CopyFcn'});
      mask Help: helpview(mapfilelocation('dspblks'), 'dspdifferentiatorfilter')
      mask Display: disp('Differentiator');
  Math Function : Math  Operator=square  SaturateOnIntegerOverflow=on
  Product1 : Product  RndMeth=Zero
  Ref. sat.1 : Saturate  UpperLimit=inf  LowerLimit=0
  Subtract : Sum  Inputs=+-
  Tref : Outport
  wires:
  Math Function/1 -> Product1/1
  Constant2/1 -> Product1/2
  wm/1 -> Math Function/1, Differentiator Filter/1(In), 1\ib1/1
  Ref. sat.1/1 -> Tref/1
  Differentiator Filter/1(Out) -> 1\ib2/1
  1\ib1/1 -> Add/2
  Product1/1 -> Subtract/1
  1\ib2/1 -> Add/1
  Subtract/1 -> Ref. sat.1/1
  Add/1 -> Subtract/2

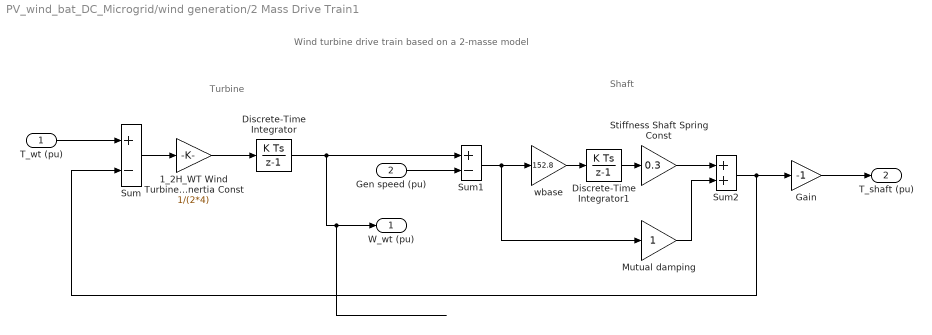
== system PV_wind_bat_DC_Microgrid/wind generation/2 Mass Drive Train1 ==
  note: Wind turbine drive train based on a 2-masse model
  note: Turbine
  note: Shaft
  T_wt (pu) : Inport
  Gen speed (pu) : Inport  Port=2
  1_2H_WT Wind Turbine Inertia Const : Gain  Gain=1/(2*4)  SaturateOnIntegerOverflow=on  OutDataTypeStr=Inherit: Same as input  ParamDataTypeStr=Inherit: Same as input
  Discrete-Time Integrator : DiscreteIntegrator  InitialCondition=1  SampleTime=20e-6  ICPrevOutput=DiscIntNeverNeededParam  ICPrevScaledInput=DiscIntNeverNeededParam
  Discrete-Time Integrator1 : DiscreteIntegrator  InitialCondition=1/0.3  SampleTime=20e-6  UpperSaturationLimit=4  LowerSaturationLimit=-4  ICPrevOutput=DiscIntNeverNeededParam  ICPrevScaledInput=DiscIntNeverNeededParam
  Gain : Gain  Gain=-1  SaturateOnIntegerOverflow=on  OutDataTypeStr=Inherit: Same as input  ParamDataTypeStr=Inherit: Same as input
  Mutual damping : Gain  SaturateOnIntegerOverflow=on  OutDataTypeStr=Inherit: Same as input  ParamDataTypeStr=Inherit: Same as input
  Stiffness Shaft Spring Const : Gain  Gain=0.3  SaturateOnIntegerOverflow=on  OutDataTypeStr=Inherit: Same as input  ParamDataTypeStr=Inherit: Same as input
  Sum : Sum  Inputs=+-  SaturateOnIntegerOverflow=on  InputSameDT=on  OutDataTypeStr=Inherit: Same as first input
  Sum1 : Sum  Inputs=+-  SaturateOnIntegerOverflow=on  InputSameDT=on  OutDataTypeStr=Inherit: Same as first input
  Sum2 : Sum  SaturateOnIntegerOverflow=on  InputSameDT=on  OutDataTypeStr=Inherit: Same as first input
  wbase : Gain  Gain=152.8  SaturateOnIntegerOverflow=on  OutDataTypeStr=Inherit: Same as input  ParamDataTypeStr=Inherit: Same as input
  W_wt (pu) : Outport
  T_shaft (pu) : Outport  Port=2
  wires:
  T_wt (pu)/1 -> Sum/1
  Sum2/1 -> Sum/2, Gain/1
  Mutual damping/1 -> Sum2/2
  Sum1/1 -> Mutual damping/1, wbase/1
  Gen speed (pu)/1 -> Sum1/2
  Discrete-Time Integrator/1 -> Sum1/1, W_wt (pu)/1
  1_2H_WT Wind Turbine Inertia Const/1 -> Discrete-Time Integrator/1
  Sum/1 -> 1_2H_WT Wind Turbine Inertia Const/1
  Stiffness Shaft Spring Const/1 -> Sum2/1
  Discrete-Time Integrator1/1 -> Stiffness Shaft Spring Const/1
  wbase/1 -> Discrete-Time Integrator1/1
  Gain/1 -> T_shaft (pu)/1

== system PV_wind_bat_DC_Microgrid/wind generation/Pitch_angle-controller ==
  wr1 : Inport
  0-pitch_max : Saturate  UpperLimit=45  LowerLimit=0
  Constant2 : Constant  Value=2
  "Rate Limiter   " : RateLimiter  RisingSlewLimit=2  FallingSlewLimit=-2
  Sum : Sum  Inputs=|+-  SaturateOnIntegerOverflow=on
  pitch_gain : Gain  Gain=500  SaturateOnIntegerOverflow=on  OutDataTypeStr=Inherit: Same as input  ParamDataTypeStr=Inherit: Same as input
  Pitch_angle1 : Outport
  wires:
  "Rate Limiter   "/1 -> Pitch_angle1/1
  pitch_gain/1 -> 0-pitch_max/1
  Sum/1 -> pitch_gain/1
  Constant2/1 -> Sum/2
  0-pitch_max/1 -> "Rate Limiter   "/1
  wr1/1 -> Sum/1

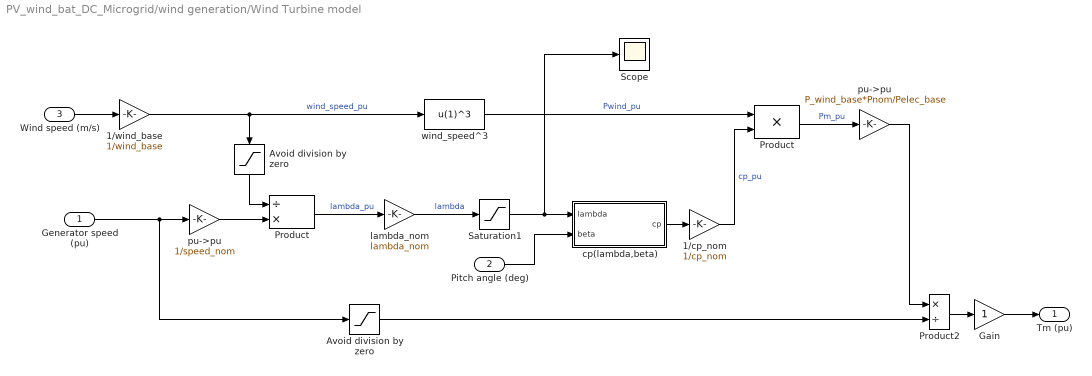
== system PV_wind_bat_DC_Microgrid/wind generation/Wind Turbine model ==
  Generator speed (pu) : Inport
  Pitch angle (deg) : Inport  Port=2
  Wind speed (m/s) : Inport  Port=3
  1/cp_nom : Gain  Gain=1/cp_nom  SaturateOnIntegerOverflow=on  OutDataTypeStr=Inherit: Same as input  ParamDataTypeStr=Inherit: Same as input
  1/wind_base : Gain  Gain=1/wind_base  SaturateOnIntegerOverflow=on  OutDataTypeStr=Inherit: Same as input  ParamDataTypeStr=Inherit: Same as input
  Avoid division by zero : Saturate  UpperLimit=1e6  LowerLimit=1e-6
  "Avoid division by zero " : Saturate  UpperLimit=1e6  LowerLimit=1e-6
  Gain : Gain  SaturateOnIntegerOverflow=on  OutDataTypeStr=Inherit: Same as input  ParamDataTypeStr=Inherit: Same as input
  Product : Product  Inputs=/*  SaturateOnIntegerOverflow=on  OutDataTypeStr=Inherit: Same as first input
  "Product " : Product  SaturateOnIntegerOverflow=on  OutDataTypeStr=Inherit: Same as first input
  Product2 : Product  Inputs=*/  SaturateOnIntegerOverflow=on  InputSameDT=on  OutDataTypeStr=Inherit: Same as first input
  Saturation1 : Saturate  UpperLimit=inf  LowerLimit=1e-6
  Scope : Scope
      settings: SaveName=ScopeData10
  cp(lambda,beta) : Subsystem
  lambda_nom : Gain  Gain=lambda_nom  SaturateOnIntegerOverflow=on  OutDataTypeStr=Inherit: Same as input  ParamDataTypeStr=Inherit: Same as input
  pu->pu : Gain  Gain=P_wind_base*Pnom/Pelec_base  SaturateOnIntegerOverflow=on  OutDataTypeStr=Inherit: Same as input  ParamDataTypeStr=Inherit: Same as input
  "pu->pu " : Gain  Gain=1/speed_nom  SaturateOnIntegerOverflow=on  OutDataTypeStr=Inherit: Same as input  ParamDataTypeStr=Inherit: Same as input
  wind_speed^3 : Fcn  Expr=u(1)^3
  Tm (pu) : Outport
  wires:
  Pitch angle (deg)/1 -> cp(lambda,beta)/2(beta)
  pu->pu/1 -> Product2/1
  cp(lambda,beta)/1(cp) -> 1/cp_nom/1
  wind_speed^3/1 -> "Product "/1  "Pwind_pu"
  Product2/1 -> Gain/1
  Avoid division by zero/1 -> Product2/2
  Wind speed (m/s)/1 -> 1/wind_base/1
  Gain/1 -> Tm (pu)/1
  Generator speed (pu)/1 -> Avoid division by zero/1, "pu->pu "/1
  "Product "/1 -> pu->pu/1  "Pm_pu"
  lambda_nom/1 -> Saturation1/1  "lambda"
  1/cp_nom/1 -> "Product "/2  "cp_pu"
  Saturation1/1 -> cp(lambda,beta)/1(lambda), Scope/1
  Product/1 -> lambda_nom/1  "lambda_pu"
  1/wind_base/1 -> wind_speed^3/1, "Avoid division by zero "/1  "wind_speed_pu"
  "Avoid division by zero "/1 -> Product/1
  "pu->pu "/1 -> Product/2

== system PV_wind_bat_DC_Microgrid/Wind-MPPT/Torque reference 1/Differentiator Filter ==
  In : Inport
  Generated Filter Block : Subsystem  Tag=FilterWizardSubSystem
      settings: ErrorFcn=dspFilterRealizedInBasicElemsAlgLoopErrFcnCallback
  Out : Outport
  wires:
  Generated Filter Block/1(Output) -> Out/1
  In/1 -> Generated Filter Block/1(Input)

== system PV_wind_bat_DC_Microgrid/wind generation/Wind Turbine model/cp(lambda,beta) ==
  lambda : Inport
  beta : Inport  Port=2
  Fcn : Fcn  Expr=1/(1/(u[1]+0.08*u[2])-0.035/(u[2]^3+1))
  Fcn1 : Fcn  Expr=c1*(c2/u[2]-c3*u[3]-c4)*exp(-c5/u[2])+c6*u[1]
  Mux : Mux  Inputs=2
  Mux1 : Mux  Inputs=3
  cp : Outport
  wires:
  Fcn/1 -> Mux1/2  "lambda_i"
  Fcn1/1 -> cp/1
  lambda/1 -> Mux1/1, Mux/1
  Mux1/1 -> Fcn1/1
  beta/1 -> Mux1/3, Mux/2
  Mux/1 -> Fcn/1
